simulink model "task3"  (R2015b)
settings: Solver=ode3  StartTime=0.0  StopTime=30  RelTol=1e-3
libraries: simulink x12, legoev3lib x6, simulink_extras x3, dspsigops x3
settings Model: SimulationMode=external  ExtModeTrigDuration=2  Creator=s079  LastModifiedBy=s079
settings OptimizationCC: DefaultParameterBehavior=Inlined  OptimizeModelRefInitCode=on  LifeSpan=1
settings HardwareCC: ProdBitPerPointer=32  ProdLargestAtomicInteger=Long  ProdWordSize=32  ProdHWDeviceType=ARM Compatible->ARM 9
settings RTWCC: SystemTargetFile=realtime.tlc  GenerateMakefile=off  TemplateMakefile=realtime.tmf  Description=Run on Target Hardware  RTWVerbose=off
settings STFCustomTargetCC: TargetLibSuffix=.a  GenerateSampleERTMain=on  ConcurrentExecutionCompliant=off  GeneratePreprocessorConditionals=Use local settings  ERTCustomFileBanners=on  SupportNonInlinedSFcns=off  SupportVariableSizeSignals=on  MATLABClassNameForMDSCustomization=Simulink.SoftwareTarget.ERTCustomization  CPPClassGenCompliant=off  GRTInterface=off  SystemTargetFile=realtime.tlc
settings ERTTargetCC: GenerateSampleERTMain=on  ParMdlRefBuildCompliant=off  CompOptLevelCompliant=off  ConcurrentExecutionCompliant=off  CombineOutputUpdateFcns=off  ERTFirstTimeCompliant=off  SupportContinuousTime=on  SupportVariableSizeSignals=on  ModelStepFunctionPrototypeControlCompliant=off  CPPClassGenCompliant=off  UseToolchainInfoCompliant=off  ERTSrcFileBannerTemplate=realtime_code_template.cgt  ERTHdrFileBannerTemplate=realtime_code_template.cgt  ERTDataSrcFileTemplate=realtime_code_template.cgt  ERTDataHdrFileTemplate=realtime_code_template.cgt  ERTCustomFileTemplate=realtime_file_process.tlc

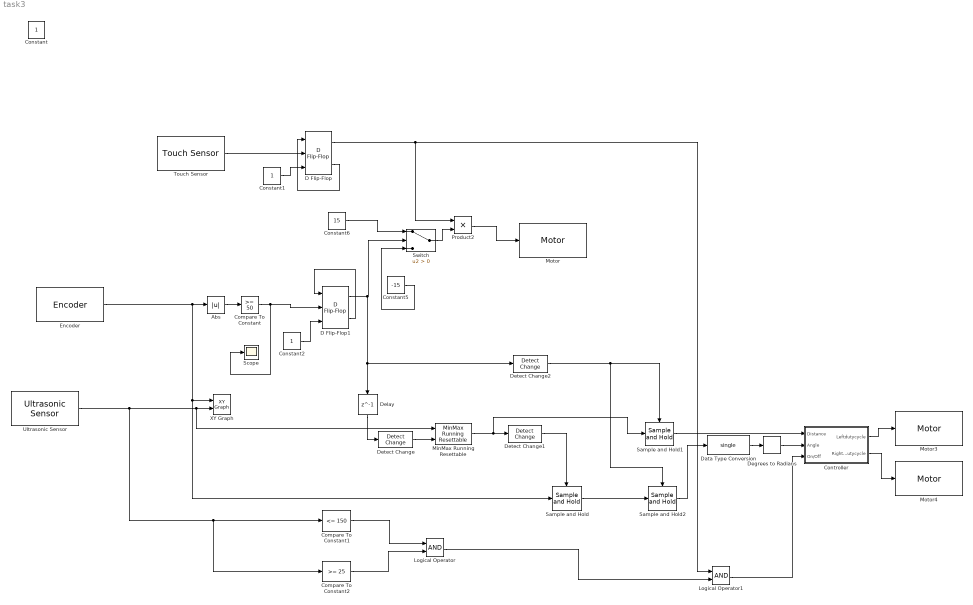
== system task3 ==
  Abs : Abs
  Compare To Constant : simulink/Logic and Bit Operations/Compare To Constant  relop=>=  const=50  OutDataTypeStr=boolean
  Compare To Constant1 : simulink/Logic and Bit Operations/Compare To Constant  relop=<=  const=150  OutDataTypeStr=boolean
  Compare To Constant2 : simulink/Logic and Bit Operations/Compare To Constant  relop=>=  const=25  OutDataTypeStr=boolean
  Constant1 : Constant
  Constant2 : Constant
  Constant5 : Constant  Value=-15
  Constant6 : Constant  Value=15
  Controller : Subsystem
  D Flip-Flop : simulink_extras/Flip Flops/D Flip-Flop
  D Flip-Flop1 : simulink_extras/Flip Flops/D Flip-Flop
  Data Type Conversion : DataTypeConversion  OutDataTypeStr=single
  Degrees to Radians : simulink_extras/Transformations/Degrees to Radians
  Delay : Delay  DelayLength=1
  Detect Change : simulink/Logic and Bit Operations/Detect Change  vinit=0  InputProcessing=Inherited  OutDataTypeStr=boolean
  Detect Change1 : simulink/Logic and Bit Operations/Detect Change  vinit=0  InputProcessing=Inherited  OutDataTypeStr=boolean
  Detect Change2 : simulink/Logic and Bit Operations/Detect Change  vinit=0  InputProcessing=Inherited  OutDataTypeStr=boolean
  Encoder : legoev3lib/Encoder  portNumber=D  opMode=No reset  sampleTime=0.01
  Logical Operator : Logic  AllPortsSameDT=off  OutDataTypeStr=boolean
  Logical Operator1 : Logic  AllPortsSameDT=off  OutDataTypeStr=boolean
  MinMax Running Resettable : simulink/Math Operations/MinMax Running Resettable  Function=min  vinit=256
  Motor : legoev3lib/Motor  sportNumber=D  sstopAction=Brake
  Motor3 : legoev3lib/Motor  sportNumber=A  sstopAction=Brake
  Motor4 : legoev3lib/Motor  sportNumber=B  sstopAction=Brake
  Product2 : Product
  Sample and Hold : dspsigops/Sample and Hold  trig=Rising edge  initCond=0  latchinput=off
  Sample and Hold1 : dspsigops/Sample and Hold  trig=Rising edge  initCond=0  latchinput=off
  Sample and Hold2 : dspsigops/Sample and Hold  trig=Rising edge  initCond=0  latchinput=off
  Scope : Scope
  Switch : Switch  Criteria=u2 > Threshold
  Touch Sensor : legoev3lib/Touch Sensor  portNumber=1  sampleTime=0.01
  Ultrasonic Sensor : legoev3lib/Ultrasonic Sensor  PortNumber=4  sampleTime=0.01
  XY Graph : simulink/Sinks/XY Graph  xmin=-100  xmax=100  ymin=-50  ymax=500  st=-1
  Constant : Constant  IOType=siggen
  wires:
  Touch Sensor/1 -> D Flip-Flop/2
  D Flip-Flop/2 -> D Flip-Flop/1
  Constant1/1 -> D Flip-Flop/3
  Constant2/1 -> D Flip-Flop1/3
  Abs/1 -> Compare To Constant/1
  Compare To Constant/1 -> Scope/1, D Flip-Flop1/2
  D Flip-Flop1/2 -> D Flip-Flop1/1
  Constant6/1 -> Switch/1
  Constant5/1 -> Switch/3
  D Flip-Flop1/1 -> Detect Change2/1, Delay/1, Switch/2
  Switch/1 -> Product2/2
  D Flip-Flop/1 -> Logical Operator1/1, Product2/1
  Product2/1 -> Motor/1
  Ultrasonic Sensor/1 -> Compare To Constant2/1, Compare To Constant1/1, MinMax Running Resettable/1, XY Graph/2
  Detect Change/1 -> MinMax Running Resettable/2
  MinMax Running Resettable/1 -> Sample and Hold1/1, Detect Change1/1
  Detect Change1/1 -> Sample and Hold/Trigger
  Sample and Hold/1 -> Sample and Hold2/1
  Detect Change2/1 -> Sample and Hold2/Trigger, Sample and Hold1/Trigger
  Compare To Constant1/1 -> Logical Operator/1
  Compare To Constant2/1 -> Logical Operator/2
  Sample and Hold1/1 -> Controller/1(Distance)
  Controller/1(Leftdutycycle) -> Motor3/1
  Controller/2(Rightdutycycle) -> Motor4/1
  Logical Operator/1 -> Logical Operator1/2
  Logical Operator1/1 -> Controller/3(On/Off)
  Delay/1 -> Detect Change/1
  Sample and Hold2/1 -> Data Type Conversion/1
  Encoder/1 -> Sample and Hold/1, XY Graph/1, Abs/1
  Degrees to Radians/1 -> Controller/2(Angle)
  Data Type Conversion/1 -> Degrees to Radians/1

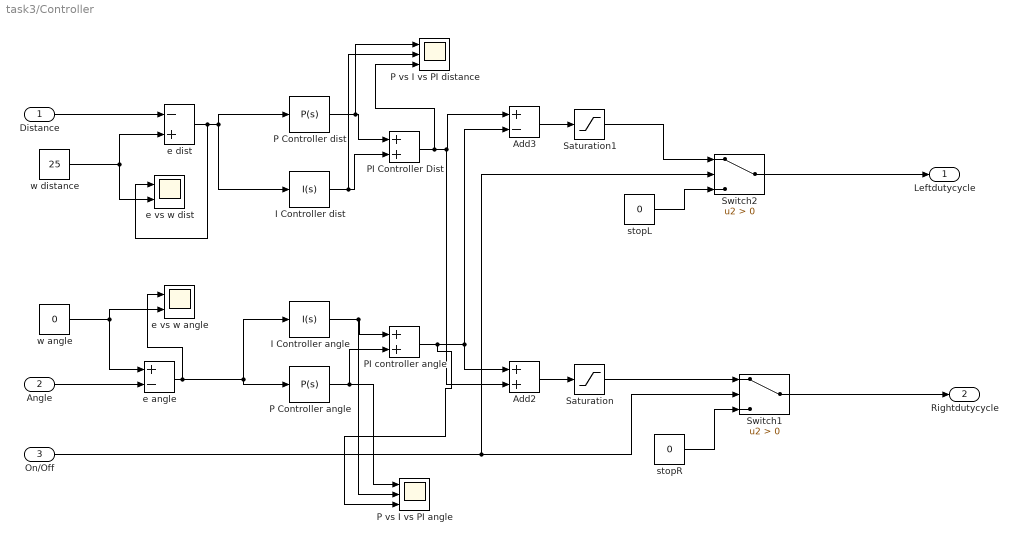
== system task3/Controller ==
  Distance : Inport
  Angle : Inport  Port=2
  On/Off : Inport  Port=3
  Add2 : Sum
  Add3 : Sum  Inputs=+-
  I Controller angle : simulink/Continuous/PID Controller  Controller=I  TimeDomain=Continuous-time  SampleTime=-1  IntegratorMethod=Forward Euler  FilterMethod=Forward Euler  Form=Parallel  UseFilter=on  ControllerParametersSource=internal  P=1  I=0.00002  D=0  N=100  InitialConditionSource=internal  InitialConditionForIntegrator=0  InitialConditionForFilter=0  ExternalReset=none  LimitOutput=off  UpperSaturationLimit=inf  LowerSaturationLimit=-inf  LinearizeAsGain=on  AntiWindupMode=none  Kb=1  TrackingMode=off  Kt=1  PParamMin=[]  PParamMax=[]  IParamMin=[]  IParamMax=[]  DParamMin=[]  DParamMax=[]  NParamMin=[]  NParamMax=[]  KbParamMin=[]  KbParamMax=[]  KtParamMin=[]  KtParamMax=[]  POutMin=[]  POutMax=[]  IOutMin=[]  IOutMax=[]  DOutMin=[]  DOutMax=[]  NOutMin=[]  NOutMax=[]  KbOutMin=[]  KbOutMax=[]  KtOutMin=[]  KtOutMax=[]  IntegratorOutMin=[]  IntegratorOutMax=[]  FilterOutMin=[]  FilterOutMax=[]  SumOutMin=[]  SumOutMax=[]  SumI1OutMin=[]  SumI1OutMax=[]  SumI2OutMin=[]  SumI2OutMax=[]  SumI3OutMin=[]  SumI3OutMax=[]  SumDOutMin=[]  SumDOutMax=[]  SaturationOutMin=[]  SaturationOutMax=[]  IntegratorContinuousStateAttributes=''  IntegratorStateMustResolveToSignalObject=off  IntegratorRTWStateStorageClass=Auto  FilterContinuousStateAttributes=''  FilterStateMustResolveToSignalObject=off  FilterRTWStateStorageClass=Auto  DifferentiatorICPrevScaledInput=0  DifferentiatorOutMin=[]  DifferentiatorOutMax=[]
  I Controller dist : simulink/Continuous/PID Controller  Controller=I  TimeDomain=Continuous-time  SampleTime=-1  IntegratorMethod=Forward Euler  FilterMethod=Forward Euler  Form=Parallel  UseFilter=on  ControllerParametersSource=internal  P=1  I=-0.05  D=0  N=100  InitialConditionSource=internal  InitialConditionForIntegrator=0  InitialConditionForFilter=0  ExternalReset=none  LimitOutput=off  UpperSaturationLimit=inf  LowerSaturationLimit=-inf  LinearizeAsGain=on  AntiWindupMode=none  Kb=1  TrackingMode=off  Kt=1  PParamMin=[]  PParamMax=[]  IParamMin=[]  IParamMax=[]  DParamMin=[]  DParamMax=[]  NParamMin=[]  NParamMax=[]  KbParamMin=[]  KbParamMax=[]  KtParamMin=[]  KtParamMax=[]  POutMin=[]  POutMax=[]  IOutMin=[]  IOutMax=[]  DOutMin=[]  DOutMax=[]  NOutMin=[]  NOutMax=[]  KbOutMin=[]  KbOutMax=[]  KtOutMin=[]  KtOutMax=[]  IntegratorOutMin=[]  IntegratorOutMax=[]  FilterOutMin=[]  FilterOutMax=[]  SumOutMin=[]  SumOutMax=[]  SumI1OutMin=[]  SumI1OutMax=[]  SumI2OutMin=[]  SumI2OutMax=[]  SumI3OutMin=[]  SumI3OutMax=[]  SumDOutMin=[]  SumDOutMax=[]  SaturationOutMin=[]  SaturationOutMax=[]  IntegratorContinuousStateAttributes=''  IntegratorStateMustResolveToSignalObject=off  IntegratorRTWStateStorageClass=Auto  FilterContinuousStateAttributes=''  FilterStateMustResolveToSignalObject=off  FilterRTWStateStorageClass=Auto  DifferentiatorICPrevScaledInput=0  DifferentiatorOutMin=[]  DifferentiatorOutMax=[]
  P Controller angle : simulink/Continuous/PID Controller  Controller=P  TimeDomain=Continuous-time  SampleTime=-1  IntegratorMethod=Forward Euler  FilterMethod=Forward Euler  Form=Parallel  UseFilter=on  ControllerParametersSource=internal  P=15  I=1  D=0  N=100  InitialConditionSource=internal  InitialConditionForIntegrator=0  InitialConditionForFilter=0  ExternalReset=none  LimitOutput=off  UpperSaturationLimit=inf  LowerSaturationLimit=-inf  LinearizeAsGain=on  AntiWindupMode=none  Kb=1  TrackingMode=off  Kt=1  PParamMin=[]  PParamMax=[]  IParamMin=[]  IParamMax=[]  DParamMin=[]  DParamMax=[]  NParamMin=[]  NParamMax=[]  KbParamMin=[]  KbParamMax=[]  KtParamMin=[]  KtParamMax=[]  POutMin=[]  POutMax=[]  IOutMin=[]  IOutMax=[]  DOutMin=[]  DOutMax=[]  NOutMin=[]  NOutMax=[]  KbOutMin=[]  KbOutMax=[]  KtOutMin=[]  KtOutMax=[]  IntegratorOutMin=[]  IntegratorOutMax=[]  FilterOutMin=[]  FilterOutMax=[]  SumOutMin=[]  SumOutMax=[]  SumI1OutMin=[]  SumI1OutMax=[]  SumI2OutMin=[]  SumI2OutMax=[]  SumI3OutMin=[]  SumI3OutMax=[]  SumDOutMin=[]  SumDOutMax=[]  SaturationOutMin=[]  SaturationOutMax=[]  IntegratorContinuousStateAttributes=''  IntegratorStateMustResolveToSignalObject=off  IntegratorRTWStateStorageClass=Auto  FilterContinuousStateAttributes=''  FilterStateMustResolveToSignalObject=off  FilterRTWStateStorageClass=Auto  DifferentiatorICPrevScaledInput=0  DifferentiatorOutMin=[]  DifferentiatorOutMax=[]
  P Controller dist : simulink/Continuous/PID Controller  Controller=P  TimeDomain=Continuous-time  SampleTime=-1  IntegratorMethod=Forward Euler  FilterMethod=Forward Euler  Form=Parallel  UseFilter=on  ControllerParametersSource=internal  P=-2  I=1  D=0  N=100  InitialConditionSource=internal  InitialConditionForIntegrator=0  InitialConditionForFilter=0  ExternalReset=none  LimitOutput=off  UpperSaturationLimit=inf  LowerSaturationLimit=-inf  LinearizeAsGain=on  AntiWindupMode=none  Kb=1  TrackingMode=off  Kt=1  PParamMin=[]  PParamMax=[]  IParamMin=[]  IParamMax=[]  DParamMin=[]  DParamMax=[]  NParamMin=[]  NParamMax=[]  KbParamMin=[]  KbParamMax=[]  KtParamMin=[]  KtParamMax=[]  POutMin=[]  POutMax=[]  IOutMin=[]  IOutMax=[]  DOutMin=[]  DOutMax=[]  NOutMin=[]  NOutMax=[]  KbOutMin=[]  KbOutMax=[]  KtOutMin=[]  KtOutMax=[]  IntegratorOutMin=[]  IntegratorOutMax=[]  FilterOutMin=[]  FilterOutMax=[]  SumOutMin=[]  SumOutMax=[]  SumI1OutMin=[]  SumI1OutMax=[]  SumI2OutMin=[]  SumI2OutMax=[]  SumI3OutMin=[]  SumI3OutMax=[]  SumDOutMin=[]  SumDOutMax=[]  SaturationOutMin=[]  SaturationOutMax=[]  IntegratorContinuousStateAttributes=''  IntegratorStateMustResolveToSignalObject=off  IntegratorRTWStateStorageClass=Auto  FilterContinuousStateAttributes=''  FilterStateMustResolveToSignalObject=off  FilterRTWStateStorageClass=Auto  DifferentiatorICPrevScaledInput=0  DifferentiatorOutMin=[]  DifferentiatorOutMax=[]
  P vs I vs PI angle : Scope  NumInputPorts=3
  P vs I vs PI distance : Scope  NumInputPorts=3
  PI Controller Dist : Sum
  PI controller angle : Sum
  Saturation : Saturate  UpperLimit=100  LowerLimit=-100
  Saturation1 : Saturate  UpperLimit=100  LowerLimit=-100
  Switch1 : Switch  Criteria=u2 > Threshold
  Switch2 : Switch  Criteria=u2 > Threshold
  e angle : Sum  Inputs=+-
  e dist : Sum  Inputs=-+
  e vs w angle : Scope  NumInputPorts=2
  e vs w dist : Scope  NumInputPorts=2
  stopL : Constant  Value=0
  stopR : Constant  Value=0
  w angle : Constant  Value=0
  w distance : Constant  Value=25
  Leftdutycycle : Outport
  Rightdutycycle : Outport  Port=2
  wires:
  Distance/1 -> e dist/1
  e dist/1 -> e vs w dist/1, P Controller dist/1, I Controller dist/1
  Add3/1 -> Saturation1/1
  Add2/1 -> Saturation/1
  P Controller dist/1 -> P vs I vs PI distance/1, PI Controller Dist/1
  I Controller dist/1 -> P vs I vs PI distance/2, PI Controller Dist/2
  I Controller angle/1 -> P vs I vs PI angle/2, PI controller angle/1
  P Controller angle/1 -> P vs I vs PI angle/1, PI controller angle/2
  PI controller angle/1 -> P vs I vs PI angle/3, Add3/2, Add2/1
  PI Controller Dist/1 -> P vs I vs PI distance/3, Add3/1, Add2/2
  w distance/1 -> e dist/2, e vs w dist/2
  Angle/1 -> e angle/2
  e angle/1 -> e vs w angle/1, I Controller angle/1, P Controller angle/1
  w angle/1 -> e angle/1, e vs w angle/2
  stopL/1 -> Switch2/3
  Saturation1/1 -> Switch2/1
  Switch2/1 -> Leftdutycycle/1
  stopR/1 -> Switch1/3
  Saturation/1 -> Switch1/1
  Switch1/1 -> Rightdutycycle/1
  On/Off/1 -> Switch2/2, Switch1/2
